simulink model "npsauv_no_converter"  (R2017a)
settings: Solver=VariableStepAuto  StartTime=0.0  StopTime=300  FixedStep=0.5  RelTol=1e-3
libraries: simulink x1
settings Model: Creator=admin  LastModifiedBy=admin

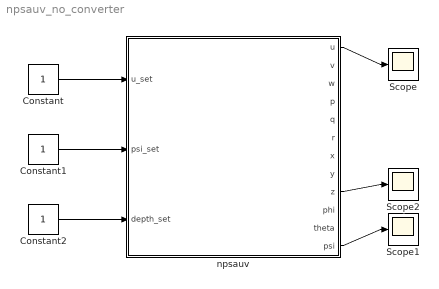
== system npsauv_no_converter ==
  Constant : Constant
  Constant1 : Constant
  Constant2 : Constant
  Scope : Scope
  Scope1 : Scope
  Scope2 : Scope
  npsauv : Subsystem  mask{x_init=[0.1 0 0 0 0 0 0 0 0 0 0 0]}
      mask prompts: x_init "initial states: [u v w p q r x y z phi theta psi]"
  wires:
  Constant/1 -> npsauv/1(u_set)
  Constant1/1 -> npsauv/2(psi_set)
  Constant2/1 -> npsauv/3(depth_set)
  npsauv/1(u) -> Scope/1
  npsauv/12(psi) -> Scope1/1
  npsauv/9(z) -> Scope2/1

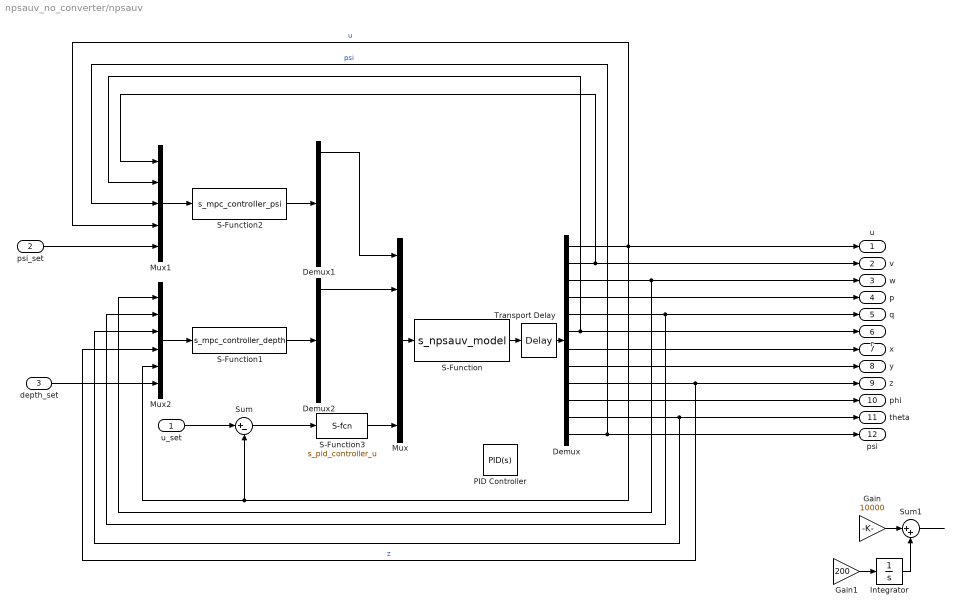
== system npsauv_no_converter/npsauv ==
  u_set : Inport
  psi_set : Inport  Port=2
  depth_set : Inport  Port=3
  Demux : Demux  Outputs=12
  Demux1 : Demux  Outputs=5
  Demux2 : Demux  Outputs=5
  Gain : Gain  Gain=10000
  Gain1 : Gain  Gain=200
  Integrator : Integrator  LimitOutput=on  UpperSaturationLimit=50  LowerSaturationLimit=-50
  Mux : Mux  Inputs=6
  Mux1 : Mux  Inputs=5
  Mux2 : Mux  Inputs=6
  PID Controller : simulink/Continuous/PID Controller  Controller=PID  TimeDomain=Continuous-time  SampleTime=-1  IntegratorMethod=Forward Euler  FilterMethod=Forward Euler  Form=Parallel  UseFilter=on  ControllerParametersSource=internal  P=5000  I=200  D=0  N=100  InitialConditionSource=internal  InitialConditionForIntegrator=0  InitialConditionForFilter=0  ExternalReset=none  LimitOutput=off  UpperSaturationLimit=inf  LowerSaturationLimit=-inf  LinearizeAsGain=on  AntiWindupMode=none  Kb=1  TrackingMode=off  Kt=1  PParamMin=[]  PParamMax=[]  IParamMin=[]  IParamMax=[]  DParamMin=[]  DParamMax=[]  NParamMin=[]  NParamMax=[]  KbParamMin=[]  KbParamMax=[]  KtParamMin=[]  KtParamMax=[]  POutMin=[]  POutMax=[]  IOutMin=[]  IOutMax=[]  DOutMin=[]  DOutMax=[]  NOutMin=[]  NOutMax=[]  KbOutMin=[]  KbOutMax=[]  KtOutMin=[]  KtOutMax=[]  IntegratorOutMin=[]  IntegratorOutMax=[]  FilterOutMin=[]  FilterOutMax=[]  SumOutMin=[]  SumOutMax=[]  SumI1OutMin=[]  SumI1OutMax=[]  SumI2OutMin=[]  SumI2OutMax=[]  SumI3OutMin=[]  SumI3OutMax=[]  SumDOutMin=[]  SumDOutMax=[]  SaturationOutMin=[]  SaturationOutMax=[]  IntegratorContinuousStateAttributes=''  IntegratorStateMustResolveToSignalObject=off  IntegratorRTWStateStorageClass=Auto  FilterContinuousStateAttributes=''  FilterStateMustResolveToSignalObject=off  FilterRTWStateStorageClass=Auto  DifferentiatorICPrevScaledInput=0  DifferentiatorOutMin=[]  DifferentiatorOutMax=[]  InitialConditionSetting=State (most efficient)
  S-Function : S-Function  FunctionName=s_npsauv_model  Parameters=x_init  SFunctionDeploymentMode=off  EnableBusSupport=off
  S-Function1 : S-Function  FunctionName=s_mpc_controller_depth  SFunctionDeploymentMode=off  EnableBusSupport=off
  S-Function2 : S-Function  FunctionName=s_mpc_controller_psi  SFunctionDeploymentMode=off  EnableBusSupport=off
  S-Function3 : S-Function  FunctionName=s_pid_controller_u  SFunctionDeploymentMode=off  EnableBusSupport=off
  Sum : Sum  Inputs=|+-
  Sum1 : Sum  Inputs=|++
  Transport Delay : TransportDelay  DelayTime=0.01
  u : Outport
  v : Outport  Port=2
  w : Outport  Port=3
  p : Outport  Port=4
  q : Outport  Port=5
  r : Outport  Port=6
  x : Outport  Port=7
  y : Outport  Port=8
  z : Outport  Port=9
  phi : Outport  Port=10
  theta : Outport  Port=11
  psi : Outport  Port=12
  wires:
  Demux/9 -> z/1, Mux2/4  "z"
  Mux/1 -> S-Function/1
  Demux2/1 -> Mux/2
  Demux/5 -> Mux2/2, q/1
  depth_set/1 -> Mux2/6
  Demux/11 -> theta/1, Mux2/3
  Mux2/1 -> S-Function1/1
  S-Function1/1 -> Demux2/1
  Demux/6 -> r/1, Mux1/2
  Demux/1 -> u/1, Mux2/5, Sum/2, Mux1/4  "u"
  u_set/1 -> Sum/1
  Demux/12 -> psi/1, Mux1/3  "psi"
  Mux1/1 -> S-Function2/1
  Demux/2 -> Mux1/1, v/1
  Demux1/1 -> Mux/1
  Demux/3 -> Mux2/1, w/1
  S-Function2/1 -> Demux1/1
  psi_set/1 -> Mux1/5
  Demux/4 -> p/1
  Demux/7 -> x/1
  Demux/8 -> y/1
  Demux/10 -> phi/1
  Integrator/1 -> Sum1/2
  Gain1/1 -> Integrator/1
  Sum1/1 -> ?
  ? -> Gain1/1, Gain/1
  Gain/1 -> Sum1/1
  S-Function3/1 -> Mux/6
  Sum/1 -> S-Function3/1
  S-Function/1 -> Transport Delay/1
  Transport Delay/1 -> Demux/1
